simulink model "TestNozzleChoked"  (R2012b)
settings: Solver=ode45  StartTime=0.0  StopTime=10.0  RelTol=1e-3
settings Model: Creator=tlavelle  LastModifiedBy=tlavelle

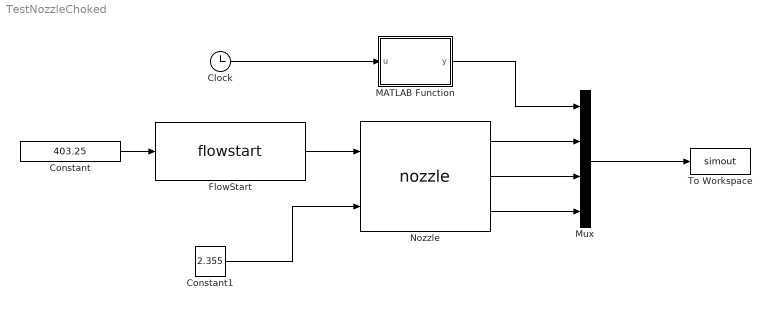
== system TestNozzleChoked ==
  Clock : Clock
  Constant : Constant  Value=403.25
  Constant1 : Constant  Value=2.355
  FlowStart : M-S-Function  FunctionName=flowstart  Parameters=Tt,Pt,comp1,comp2,comp3,comp4,comp5,comp6  mask{Tt=533.30, Pt=6.47, comp1=1, comp2=0, comp3=0, comp4=0, comp5=0, comp6=0}
      mask prompts: Tt "Exit Temperature"; Pt "Exit Pressure"
      mask Display:
      | color('red'); port_label('input',1,'Flow')
      | color('red'); port_label('output',1,'Flow Out')
  MATLAB Function : MATLAB Function  TreatAsAtomicUnit=on
  Mux : Mux
  Nozzle : M-S-Function  FunctionName=nozzle  Parameters=Wdes,Cfg,Ath_in,IDes  mask{Wdes=366.66, Cfg=.9975, Ath_in=2706.36, IDes=1}
      mask prompts: Wdes "Design Flow"; Ath_in "Throat input area"
      mask Display:
      | color('red'); port_label('input',1,'Flow In')
      | color('red'); port_label('input',2,'Ambient Pressure')
      | 
      | color('Blue'); port_label('output',1,'Flow Error')
      | color('green'); port_label('output',2,'Fg')
  To Workspace : ToWorkspace  VariableName=simout  SampleTime=-1  SaveFormat=Timeseries
  wires:
  Constant/1 -> FlowStart/1
  FlowStart/1 -> Nozzle/1
  Constant1/1 -> Nozzle/2
  Clock/1 -> MATLAB Function/1(u)
  MATLAB Function/1(y) -> Mux/1
  Nozzle/1 -> Mux/2
  Nozzle/2 -> Mux/3
  Nozzle/3 -> Mux/4
  Mux/1 -> To Workspace/1

== matlab function TestNozzleChoked/MATLAB Function ==
  data: u input; y output
function y = fcn(u)
%#codegen
eml.extrinsic('set_param');
if u < 3
   set_param('TestNozzleChoked/Nozzle','IDes','0');
elseif u< 6 
   set_param('TestNozzleChoked/Nozzle','IDes','1'); 
else 
   set_param('TestNozzleChoked/Nozzle','IDes','2'); 
end    
y = u;
